simulink model "Simulation"  (R2018a)
settings: Solver=VariableStepAuto  StartTime=0.0  StopTime=10  FixedStep=1e-6  MaxStep=Tsc  RelTol=1e-3  EnableMultiTasking=on
InitFcn:
  | clc
  | close all
  | clear all
  | 
  | %Vector-space-decomposition transform (2)
  | D = 2/6*[cos(0) cos(1*pi/3) cos(2*pi/3) cos(3*pi/3) cos(4*pi/3) cos(5*pi/3);
  |         sin(0) sin(1*pi/3) sin(2*pi/3) sin(3*pi/3) sin(4*pi/3) sin(5*pi/3);
  |         cos(2*0) cos(2*pi/3) cos(4*pi/3) cos(6*pi/3) cos(8*pi/3) cos(10*pi/3);
  |         sin(2*0) sin(2*pi/3) sin(4*pi/3) sin(6*pi/3) sin(8*pi/3) sin(10*pi/3);
  |         1/2 1/2  1/2 1/2 1/2 1/2;
  |         1/2 -1/2 1/2 -1/2 1/2 -1/2];
  | 
  | %Control sampling period
  | Tsc = 1e-4;
  | 
  | %Parameters of six-phase induction machine (other than stator resistance):
  | P=2; %Number of machine pole pairs
  | Lm=284e-3; %alpha-beta magnetizing inductance (mH)
  | Rr=2.9; %alpha-beta rotor resistance (ohm)
  | Lls=10e-3; %alpha-beta stator leakage inductance (mH)
  | Llr=21e-3; %alpha-beta rotor leakage inductance (mH)
  | Lxy=4.52e-3; %xy stator inductance (mH)
  | L0=24.5e-3; %0- stator inductance (mH)
  | J=0.0261; %Inertia (Kg*m^2)
  | f=0.0033; %Friction coefficient (N*m*s)
  | Ls = Lls+Lm; Lr = Llr+Lm;  %alpha-beta self-inductances (mH)
undefined symbols (not defined in the file): DiscIntNeverNeededParam
libraries: powerlib x37, simulink x20, simulink_extras x7
(part 1 of 3)
settings Model: Creator=ayman.abdel-khalik  LastModifiedBy=agyepes
settings DataIOCC: LimitDataPoints=on  SaveFormat=Array
settings OptimizationCC: LifeSpan=inf
settings DebuggingCC: SolverPrmCheckMsg=warning  AllowSymbolicDim=off  SFUnexpectedBacktrackingDiag=warning  SFNoUnconditionalDefaultTransitionDiag=warning  SFExecutionAtInitializationDiag=none
settings HardwareCC: ProdBitPerPointer=32  ProdBitPerSizeT=32  ProdBitPerPtrDiffT=32  ProdLargestAtomicFloat=None  ProdIntDivRoundTo=Undefined  ProdEndianess=Unspecified  ProdWordSize=32  ProdHWDeviceType=32-bit Generic
settings ModelReferenceCC: PropagateSignalLabelsOutOfModel=off
settings CodeAppCC: StateflowObjectComments=on
settings GRTTargetCC: TargetLangStandard=C89/C90 (ANSI)
settings ConfigComp: CovMetricSettings=dw  CovSaveCumulativeToWorkspaceVar=on  CovSaveSingleToWorkspaceVar=on  CovExternalEMLEnable=off  CovSFcnEnable=off
settings SimscapeCC: SimscapeNormalizeSystem=off

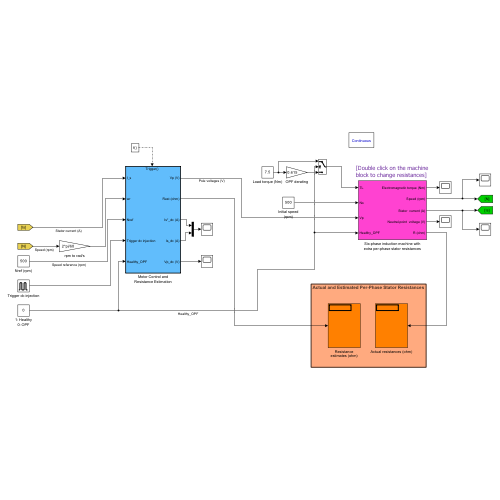
[thumbnail: Simulink's stored preview of the top-level diagram]
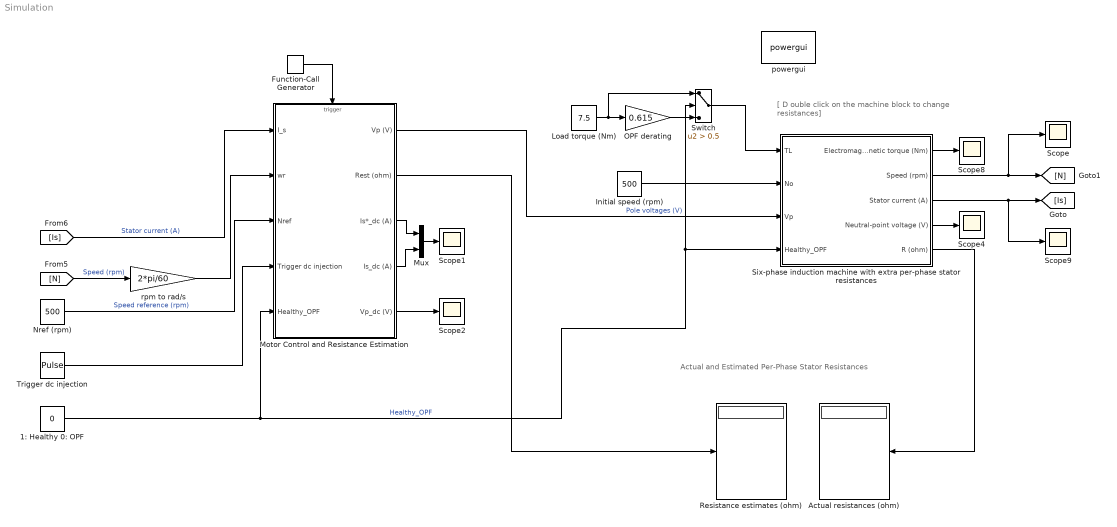
== system Simulation ==
  note: Actual and Estimated Per-Phase Stator Resistances
  note: [ D ouble click on the machine
      | block to change resistances]
  1: Healthy 0: OPF : Constant  Value=0
  Actual resistances (ohm) : Display
  Function-Call Generator : simulink/Ports & Subsystems/Function-Call Generator  sample_time=Tsc  numberOfIterations=1
  Initial speed (rpm) : Constant  Value=500
  Load torque (Nm) : Constant  Value=7.5
  Motor Control and Resistance Estimation : Subsystem
  Mux : Mux  Inputs=2
  Nref (rpm) : Constant  Value=500
  OPF derating : Gain  Gain=0.615
  Resistance estimates (ohm) : Display
  Scope{,1..2,4,8..9} (6 alike) : Scope
  Six-phase induction machine with extra per-phase stator resistances : Subsystem  mask{Radd=[3.15 5.1 2.15 4.4 0.2 0.05], Rs=4.4, Rr=Rr, Lm=Lm, Ls=Ls, Lr=Lr}
      mask prompts: Radd "Additional per-phase resistances [0-100] (ohm)"; Rs "Nominal stator resistance (ohm)"; Rr "Rotor resistance"; Lm "Alpha-beta magnetizing inductance"; Ls "Alpha-beta stator self-inductance"; Lr "Alpha-beta rotor self-inductance"
      mask init:
      | %In absence of extra resistances, the stator resistance is equal in all VSD
      | %subspaces:
      | Rxy = Rs;
      | R0 = Rs;
      | 
      | %Matrices for the machine alpha-beta equivalent circuit:
      | R1 = diag([Rs Rs Rr Rr]);
      | L1 = [Ls 0 Lm 0;
      | 	  0 Ls 0 Lm;
      | 	  Lm 0 Lr 0;
      | 	  0 Lm 0 Lr];
      | G1 = [0 0 0 0;
      |     0 0 0 0;
      |     0 0 0 1;
      |     0 0 -1 0];
      | 
      | L2=[0 0 Lm 0;
      | 	  0 0 0 Lm;
      | 	  0 0 0 0];
  Switch : Switch  Criteria=u2 > Threshold  Threshold=0.5
  Trigger dc injection : DiscretePulseGenerator  PulseType=Time based  Period=360  PhaseDelay=2
  powergui : powerlib/powergui  Priority=1  SimulationMode=Continuous  SampleTime=1e-4  frequency=60  Iterations=50  frequencyindice=0  Pbase=100e6  ErrMax=1e-4  UnitsV=kV  UnitsW=MW  buscounter=0  FunctionMessages=off  echomessages=off  EnableUseOfTLC=off  CurrentSourceSwitches=off  DisableSnubberDevices=off  DisableRonSwitches=off  DisableVfSwitches=off  DisplayEquations=off  AutomaticDiscreteSolvers=off  SolverType=Tustin/Backward Euler (TBE)  Interpol=off  ExternalGateDelay=off  methode=off  Ts=100  x0status=blocks  SPID=off  SwTol=0  HookPort=off  NonlinearTolerance=1e-4  nMaxIteration=100  ContinueOnMaxIteration=off  RestoreLinks=warning  ResistiveCurrentMeasurement=off  Frange=[0:2:500]  Ylog=off  Xlog=on  ShowGrid=off  save=off  variable=ZData  structure=0  ZoomFFT=off  StartTime=0.0  cycles=1  DisplayStyle=1  fundamental=60  FreqAxis=off  MaxFrequency=1000  frequencyindicesteady=1  RmsSteady=1  display=off
  rpm to rad/s : Gain  Gain=2*pi/60
  wires:
  [N] -> rpm to rad/s/1  "Speed (rpm)"
  [Is] -> Motor Control and Resistance Estimation/1(I_s)  "Stator current (A)"
  rpm to rad/s/1 -> Motor Control and Resistance Estimation/2(wr)
  Nref (rpm)/1 -> Motor Control and Resistance Estimation/3(Nref)  "Speed reference (rpm)"
  Motor Control and Resistance Estimation/1(Vp (V)) -> Six-phase induction machine with extra per-phase stator resistances/3(Vp)  "Pole voltages (V)"
  Motor Control and Resistance Estimation/2(Rest (ohm)) -> Resistance estimates (ohm)/1
  Trigger dc injection/1 -> Motor Control and Resistance Estimation/4(Trigger dc injection)
  Function-Call Generator/1 -> Motor Control and Resistance Estimation/Trigger
  Six-phase induction machine with extra per-phase stator resistances/2(Speed (rpm)) -> Scope/1, [N]
  Six-phase induction machine with extra per-phase stator resistances/3(Stator current (A)) -> Scope9/1, [Is]
  Switch/1 -> Six-phase induction machine with extra per-phase stator resistances/1(TL)
  Initial speed (rpm)/1 -> Six-phase induction machine with extra per-phase stator resistances/2(No)
  Six-phase induction machine with extra per-phase stator resistances/1(Electromagnetic torque (Nm)) -> Scope8/1
  Six-phase induction machine with extra per-phase stator resistances/4(Neutral-point voltage (V)) -> Scope4/1
  Six-phase induction machine with extra per-phase stator resistances/5(R (ohm)) -> Actual resistances (ohm)/1
  1: Healthy 0: OPF/1 -> Switch/2, Six-phase induction machine with extra per-phase stator resistances/4(Healthy_OPF), Motor Control and Resistance Estimation/5(Healthy_OPF)  "Healthy_OPF"
  Load torque (Nm)/1 -> Switch/1, OPF derating/1
  OPF derating/1 -> Switch/3
  Motor Control and Resistance Estimation/3(Is*_dc (A)) -> Mux/1
  Motor Control and Resistance Estimation/4(Is_dc (A)) -> Mux/2
  Mux/1 -> Scope1/1
  Motor Control and Resistance Estimation/5(Vp_dc (V)) -> Scope2/1

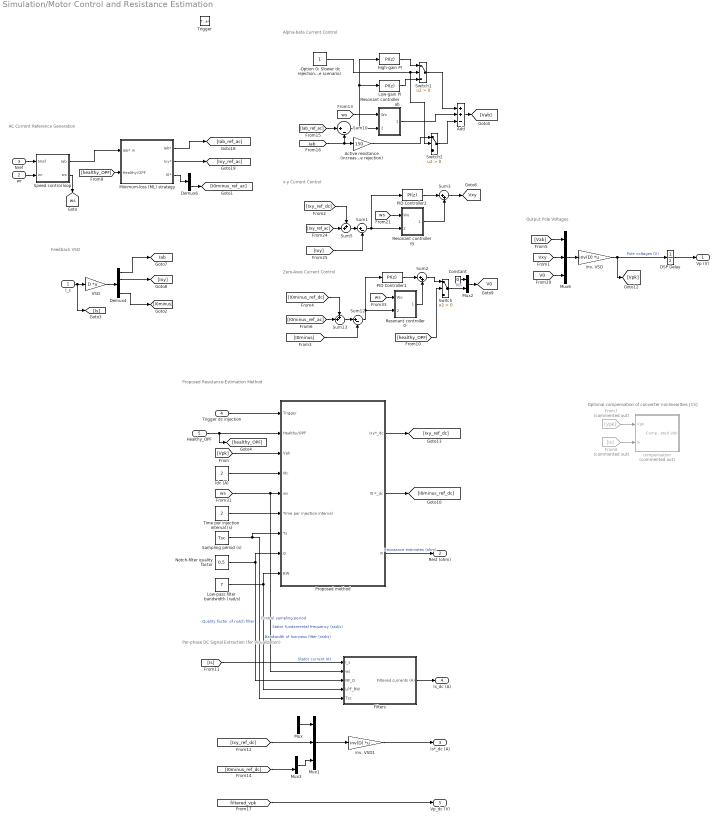
== system Simulation/Motor Control and Resistance Estimation ==
  note: Per-phase DC Signal Extraction (for Visualization)
  note: Optional compensation of converter nonlinearities [15]
  note: AC Current Reference Generation
  note: Output Pole Voltages
  note: Alpha-beta Current Control
  note: Feedback VSD
  note: x-y Current Control
  note: Zero-Axes Current Control
  note: Proposed Resistance-Estimation Method
  I_s : Inport
  wr : Inport  Port=2
  Nref : Inport  Port=3
  Trigger dc injection : Inport  Port=4
  Healthy_OPF : Inport  Port=5
  Trigger : TriggerPort  TriggerType=function-call  VariantControl=(inherit)  SampleTime=1e-4  PortDimensions=1
  "-Option 0: Slower dc rejection -Option 1: Faster dc rejection In experiments, 0 is used (worst-case scenario)" : Constant
  Active resistance (increases disturbance rejection) : Gain  Gain=150
  Add : Sum  Inputs=++-
  Constant : Constant  Value=0
  DSP Delay : UnitDelay  SampleTime=-1  HasFrameUpgradeWarning=on
  Demux4 : Demux  Outputs=[2 2 1 1 ]
  Demux6 : Demux  Outputs=2
  Filters : Subsystem
  From7 : From  Commented=on  GotoTag=Vpk
  From8 : From  Commented=on  GotoTag=Is
  High-gain PI : simulink/Continuous/PID Controller  Controller=PI  Form=Parallel  TimeDomain=Discrete-time  SampleTime=-1  IntegratorMethod=Forward Euler  ControllerParametersSource=internal  P=5  I=20000  D=0.001  N=100  UseFilter=on  TunerSelectOption=Transfer Function Based (PID Tuner App)  ZeroCross=off  InitialConditionSource=internal  InitialConditionForIntegrator=0  InitialConditionForFilter=0  DifferentiatorICPrevScaledInput=0  ExternalReset=none  TrackingMode=off  Kt=1  LimitOutput=on  UpperSaturationLimit=100  LowerSaturationLimit=-100  LinearizeAsGain=off  AntiWindupMode=clamping  Kb=1  POutMin=[]  POutMax=[]  IOutMin=[]  IOutMax=[]  DOutMin=[]  DOutMax=[]  NOutMin=[]  NOutMax=[]  SumOutMin=[]  SumOutMax=[]  SaturationOutMin=[]  SaturationOutMax=[]  PParamMin=[]  PParamMax=[]  IParamMin=[]  IParamMax=[]  DParamMin=[]  DParamMax=[]  NParamMin=[]  NParamMax=[]  KbParamMin=[]  KbParamMax=[]  KtParamMin=[]  KtParamMax=[]  KbOutMin=[]  KbOutMax=[]  KtOutMin=[]  KtOutMax=[]  IntegratorOutMin=[]  IntegratorOutMax=[]  FilterOutMin=[]  FilterOutMax=[]  SumI1OutMin=[]  SumI1OutMax=[]  SumI2OutMin=[]  SumI2OutMax=[]  SumI3OutMin=[]  SumI3OutMax=[]  SumDOutMin=[]  SumDOutMax=[]  DifferentiatorOutMin=[]  DifferentiatorOutMax=[]  FilterDiffOutCoefMin=[]  FilterDiffOutCoefMax=[]  ReciprocalOutMin=[]  ReciprocalOutMax=[]  SumDenOutMin=[]  SumDenOutMax=[]  SumNumOutMin=[]  SumNumOutMax=[]  DivideOutMin=[]  DivideOutMax=[]  IntegratorContinuousStateAttributes=''  IntegratorStateMustResolveToSignalObject=off  IntegratorRTWStateStorageClass=Auto  FilterContinuousStateAttributes=''  FilterStateMustResolveToSignalObject=off  FilterRTWStateStorageClass=Auto
  Idc (A) : Constant  Value=2
  Low-gain PI : simulink/Continuous/PID Controller  Controller=PI  Form=Parallel  TimeDomain=Discrete-time  SampleTime=-1  IntegratorMethod=Forward Euler  ControllerParametersSource=internal  P=2.6  I=670  D=0.001  N=100  UseFilter=on  TunerSelectOption=Transfer Function Based (PID Tuner App)  ZeroCross=off  InitialConditionSource=internal  InitialConditionForIntegrator=0  InitialConditionForFilter=0  DifferentiatorICPrevScaledInput=0  ExternalReset=none  TrackingMode=off  Kt=1  LimitOutput=on  UpperSaturationLimit=100  LowerSaturationLimit=-100  LinearizeAsGain=off  AntiWindupMode=clamping  Kb=1  POutMin=[]  POutMax=[]  IOutMin=[]  IOutMax=[]  DOutMin=[]  DOutMax=[]  NOutMin=[]  NOutMax=[]  SumOutMin=[]  SumOutMax=[]  SaturationOutMin=[]  SaturationOutMax=[]  PParamMin=[]  PParamMax=[]  IParamMin=[]  IParamMax=[]  DParamMin=[]  DParamMax=[]  NParamMin=[]  NParamMax=[]  KbParamMin=[]  KbParamMax=[]  KtParamMin=[]  KtParamMax=[]  KbOutMin=[]  KbOutMax=[]  KtOutMin=[]  KtOutMax=[]  IntegratorOutMin=[]  IntegratorOutMax=[]  FilterOutMin=[]  FilterOutMax=[]  SumI1OutMin=[]  SumI1OutMax=[]  SumI2OutMin=[]  SumI2OutMax=[]  SumI3OutMin=[]  SumI3OutMax=[]  SumDOutMin=[]  SumDOutMax=[]  DifferentiatorOutMin=[]  DifferentiatorOutMax=[]  FilterDiffOutCoefMin=[]  FilterDiffOutCoefMax=[]  ReciprocalOutMin=[]  ReciprocalOutMax=[]  SumDenOutMin=[]  SumDenOutMax=[]  SumNumOutMin=[]  SumNumOutMax=[]  DivideOutMin=[]  DivideOutMax=[]  IntegratorContinuousStateAttributes=''  IntegratorStateMustResolveToSignalObject=off  IntegratorRTWStateStorageClass=Auto  FilterContinuousStateAttributes=''  FilterStateMustResolveToSignalObject=off  FilterRTWStateStorageClass=Auto
  Low-pass filter bandwidth (rad/s) : Constant  Value=7
  Minimum-loss (ML) strategy : Subsystem
  Mux : Mux  Inputs=2
  Mux1 : Mux  Inputs=3
  Mux2 : Mux  Inputs=2
  Mux3 : Mux  Inputs=2
  Mux6 : Mux  Inputs=3
  Notch-filter quality factor : Constant  Value=0.5
  PID Controller1 : simulink/Continuous/PID Controller  Controller=PI  Form=Parallel  TimeDomain=Discrete-time  SampleTime=-1  IntegratorMethod=Forward Euler  ControllerParametersSource=internal  P=1.6  I=670  D=0.001  N=100  UseFilter=on  TunerSelectOption=Transfer Function Based (PID Tuner App)  ZeroCross=off  InitialConditionSource=internal  InitialConditionForIntegrator=0  InitialConditionForFilter=0  DifferentiatorICPrevScaledInput=0  ExternalReset=none  TrackingMode=off  Kt=1  LimitOutput=on  UpperSaturationLimit=100  LowerSaturationLimit=-100  LinearizeAsGain=off  AntiWindupMode=clamping  Kb=1  POutMin=[]  POutMax=[]  IOutMin=[]  IOutMax=[]  DOutMin=[]  DOutMax=[]  NOutMin=[]  NOutMax=[]  SumOutMin=[]  SumOutMax=[]  SaturationOutMin=[]  SaturationOutMax=[]  PParamMin=[]  PParamMax=[]  IParamMin=[]  IParamMax=[]  DParamMin=[]  DParamMax=[]  NParamMin=[]  NParamMax=[]  KbParamMin=[]  KbParamMax=[]  KtParamMin=[]  KtParamMax=[]  KbOutMin=[]  KbOutMax=[]  KtOutMin=[]  KtOutMax=[]  IntegratorOutMin=[]  IntegratorOutMax=[]  FilterOutMin=[]  FilterOutMax=[]  SumI1OutMin=[]  SumI1OutMax=[]  SumI2OutMin=[]  SumI2OutMax=[]  SumI3OutMin=[]  SumI3OutMax=[]  SumDOutMin=[]  SumDOutMax=[]  DifferentiatorOutMin=[]  DifferentiatorOutMax=[]  FilterDiffOutCoefMin=[]  FilterDiffOutCoefMax=[]  ReciprocalOutMin=[]  ReciprocalOutMax=[]  SumDenOutMin=[]  SumDenOutMax=[]  SumNumOutMin=[]  SumNumOutMax=[]  DivideOutMin=[]  DivideOutMax=[]  IntegratorContinuousStateAttributes=''  IntegratorStateMustResolveToSignalObject=off  IntegratorRTWStateStorageClass=Auto  FilterContinuousStateAttributes=''  FilterStateMustResolveToSignalObject=off  FilterRTWStateStorageClass=Auto
  PID Controller2 : simulink/Continuous/PID Controller  Controller=PI  Form=Parallel  TimeDomain=Discrete-time  SampleTime=-1  IntegratorMethod=Forward Euler  ControllerParametersSource=internal  P=1.6  I=670  D=0.001  N=100  UseFilter=on  TunerSelectOption=Transfer Function Based (PID Tuner App)  ZeroCross=off  InitialConditionSource=internal  InitialConditionForIntegrator=0  InitialConditionForFilter=0  DifferentiatorICPrevScaledInput=0  ExternalReset=none  TrackingMode=off  Kt=1  LimitOutput=on  UpperSaturationLimit=100  LowerSaturationLimit=-100  LinearizeAsGain=off  AntiWindupMode=clamping  Kb=1  POutMin=[]  POutMax=[]  IOutMin=[]  IOutMax=[]  DOutMin=[]  DOutMax=[]  NOutMin=[]  NOutMax=[]  SumOutMin=[]  SumOutMax=[]  SaturationOutMin=[]  SaturationOutMax=[]  PParamMin=[]  PParamMax=[]  IParamMin=[]  IParamMax=[]  DParamMin=[]  DParamMax=[]  NParamMin=[]  NParamMax=[]  KbParamMin=[]  KbParamMax=[]  KtParamMin=[]  KtParamMax=[]  KbOutMin=[]  KbOutMax=[]  KtOutMin=[]  KtOutMax=[]  IntegratorOutMin=[]  IntegratorOutMax=[]  FilterOutMin=[]  FilterOutMax=[]  SumI1OutMin=[]  SumI1OutMax=[]  SumI2OutMin=[]  SumI2OutMax=[]  SumI3OutMin=[]  SumI3OutMax=[]  SumDOutMin=[]  SumDOutMax=[]  DifferentiatorOutMin=[]  DifferentiatorOutMax=[]  FilterDiffOutCoefMin=[]  FilterDiffOutCoefMax=[]  ReciprocalOutMin=[]  ReciprocalOutMax=[]  SumDenOutMin=[]  SumDenOutMax=[]  SumNumOutMin=[]  SumNumOutMax=[]  DivideOutMin=[]  DivideOutMax=[]  IntegratorContinuousStateAttributes=''  IntegratorStateMustResolveToSignalObject=off  IntegratorRTWStateStorageClass=Auto  FilterContinuousStateAttributes=''  FilterStateMustResolveToSignalObject=off  FilterRTWStateStorageClass=Auto
  Proposed method : Subsystem
  Resonant controller 0- : Subsystem
  Resonant controller ab : Subsystem
  Resonant controller xy : Subsystem
  Sampling period (s) : Constant  Value=Tsc
  Speed control loop : Subsystem
  Sum1 : Sum  Inputs=|+-
  Sum10 : Sum  Inputs=|+-
  Sum12 : Sum  Inputs=|+-
  Sum13 : Sum  Inputs=++|
  Sum2 : Sum  Inputs=|++
  Sum3 : Sum  Inputs=|++
  Sum5 : Sum  Inputs=++|
  Switch : Switch  Criteria=u2 > Threshold
  Switch1 : Switch  Criteria=u2 > Threshold
  Switch2 : Switch  Criteria=u2 > Threshold
  Time per injection interval (s) : Constant  Value=2
  VSD : Gain  Gain=D  Multiplication=Matrix(K*u)
  compensation : Subsystem  Commented=on  mask{VDC=300, TPWM=Tsc, DT0=380e-9, ton=750e-9, toff=900e-9}
      mask prompts: VDC "Dc-link voltage (V)"; TPWM "Switching period (s)"; DT0 "Dead time (s)"; ton "Turn-on time (s)"; toff "Turn-off time (s)"
      mask init:
      | DT=DT0/TPWM;
      | Dly=(toff-ton)/TPWM;
  inv. VSD : Gain  Gain=inv(D)  Multiplication=Matrix(K*u)
  inv. VSD1 : Gain  Gain=inv(D)  Multiplication=Matrix(K*u)
  Vp (V) : Outport
  Rest (ohm) : Outport  Port=2
  Is*_dc (A) : Outport  Port=3
  Is_dc (A) : Outport  Port=4
  Vp_dc (V) : Outport  Port=5
  tag scope: Iab=global, V0=global, Vxy=global, ws=global
  wires:
  [Iab] -> Active resistance (increases disturbance rejection)/1, Sum10/2
  Sum10/1 -> Low-gain PI/1, High-gain PI/1, Resonant controller ab/2(error)
  [ws] -> Resonant controller ab/1(Wo)
  Add/1 -> [Vab]
  Mux6/1 -> inv. VSD/1
  wr/1 -> Speed control loop/2(wr)
  Nref/1 -> Speed control loop/1(Nref)
  inv. VSD/1 -> DSP Delay/1, [Vpk]  "Pole voltages (V)"
  [Vxy] -> Mux6/2
  [V0] -> Mux6/3
  [Vab] -> Mux6/1
  Demux4/4 -> [I0minus]
  Demux4/2 -> [Ixy]
  I_s/1 -> [Is], VSD/1
  Demux4/1 -> [Iab]
  VSD/1 -> Demux4/1
  Speed control loop/2(ws) -> [ws]
  Speed control loop/1(Iab) -> Minimum-loss (ML) strategy/1(Iab* in)
  Demux6/2 -> [I0minus_ref_ac]
  Minimum-loss (ML) strategy/1(Iab*) -> [Iab_ref_ac]
  Minimum-loss (ML) strategy/2(Ixy*) -> [Ixy_ref_ac]
  Minimum-loss (ML) strategy/3(I0*) -> Demux6/1
  Sum5/1 -> Sum1/1
  [ws] -> Resonant controller xy/1(Wo)
  PID Controller2/1 -> Sum3/1
  [Ixy] -> Sum1/2
  [Ixy_ref_dc] -> Sum5/1
  Sum1/1 -> Resonant controller xy/2(error), PID Controller2/1
  Sum3/1 -> [Vxy]
  Mux2/1 -> [V0]
  Sum13/1 -> Sum12/1
  [I0minus_ref_dc] -> Sum13/1
  Sum12/1 -> Resonant controller 0-/2(error), PID Controller1/1
  [I0minus] -> Sum12/2
  [ws] -> Resonant controller 0-/1(Wo)
  From7/1 -> compensation/1(Vpk)
  From8/1 -> compensation/2(Is)
  [Vpk] -> Proposed method/3(Vpk)
  [Iab_ref_ac] -> Sum10/1
  Resonant controller ab/1(Vref) -> Add/2
  Resonant controller xy/1(Vref) -> Sum3/2
  PID Controller1/1 -> Sum2/1
  Resonant controller 0-/1(Vref) -> Sum2/2
  Switch/1 -> Mux2/2  "V0-"
  Healthy_OPF/1 -> [healthy_OPF], Proposed method/2(Healthy/OPF)
  Proposed method/1(Ixy*_dc) -> [Ixy_ref_dc]
  Trigger dc injection/1 -> Proposed method/1(Trigger)
  Proposed method/2(I0-*_dc) -> [I0minus_ref_dc]
  Proposed method/3("R ") -> Rest (ohm)/1  "Resistance estimates (ohm)"
  [Ixy_ref_ac] -> Sum5/2
  DSP Delay/1 -> Vp (V)/1
  [I0minus_ref_ac] -> Sum13/2
  Idc (A)/1 -> Proposed method/4(Idc)
  Time per injection interval (s)/1 -> Proposed method/6(Time per injection interval)
  [healthy_OPF] -> Minimum-loss (ML) strategy/2(Healthy/OPF)
  Constant/1 -> Mux2/1
  [healthy_OPF] -> Switch/2
  Sum2/1 -> Switch/1
  Switch1/1 -> Add/1
  Switch2/1 -> Add/3
  High-gain PI/1 -> Switch1/1
  Active resistance (increases disturbance rejection)/1 -> Switch2/1
  "-Option 0: Slower dc rejection -Option 1: Faster dc rejection In experiments, 0 is used (worst-case scenario)"/1 -> Switch2/2, Switch1/2
  Low-gain PI/1 -> Switch1/3
  [Is] -> Filters/1(I_s)  "Stator current (A)"
  [ws] -> Filters/2(ws), Proposed method/5(ws)  "Stator fundamental frequency (rad/s)"
  Notch-filter quality factor/1 -> Filters/3(NF_Q), Proposed method/8(Q)  "Quality factor of notch filter"
  Low-pass filter bandwidth (rad/s)/1 -> Filters/4(LPF_BW), Proposed method/9(BW)  "Bandwidth of low-pass filter (rad/s)"
  Sampling period (s)/1 -> Filters/5(Tsc), Proposed method/7(Ts)  "Control sampling period"
  [Ixy_ref_dc] -> Mux1/2
  Mux/1 -> Mux1/1
  Mux1/1 -> inv. VSD1/1
  [I0minus_ref_dc] -> Mux3/2
  Mux3/1 -> Mux1/3
  Filters/1(Filtered currents (A)) -> Is_dc (A)/1
  inv. VSD1/1 -> Is*_dc (A)/1
  [filtered_vpk] -> Vp_dc (V)/1

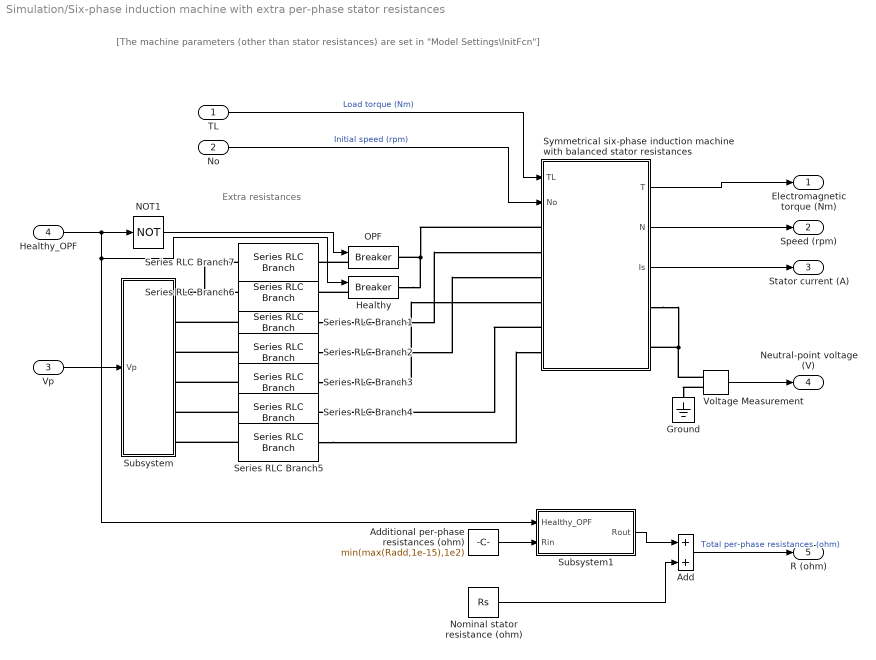
== system Simulation/Six-phase induction machine with extra per-phase stator resistances ==
  note: [The machine parameters (other than stator resistances) are set in "Model Settings\InitFcn"]
  note: Extra resistances
  TL : Inport
  No : Inport  Port=2
  Vp : Inport  Port=3
  Healthy_OPF : Inport  Port=4
  Add : Sum
  Additional per-phase resistances (ohm) : Constant  Value=min(max(Radd,1e-15),1e2)
  Ground : powerlib/Elements/Ground  LConnTagsString=a
  Healthy : powerlib/Elements/Breaker  InitialState=1  SwitchingTimes="[1/60  5/60]"  External=on  BreakerResistance=0  SnubberResistance=1e6  SnubberCapacitance=inf  Measurements=None  MoreParameters=on  NoBreakLoop=off
  NOT1 : Logic  Operator=NOT  IconShape=distinctive  AllPortsSameDT=off  OutDataTypeStr=boolean
  Nominal stator resistance (ohm) : Constant  Value=Rs
  OPF : powerlib/Elements/Breaker  InitialState=0  SwitchingTimes="[1/60  5/60]"  External=on  BreakerResistance=0  SnubberResistance=1e6  SnubberCapacitance=inf  Measurements=None  MoreParameters=on  NoBreakLoop=off
  Series RLC Branch1 : powerlib/Elements/Series RLC Branch  LConnTagsString=__new0  RConnTagsString=__new0  BranchType=R  Resistance=min(max(Radd(2),1e-15),1e2)  Inductance=1e-3  SetiL0=off  InitialCurrent=0  Capacitance=1e-6  Setx0=off  InitialVoltage=0  Measurements=None
  Series RLC Branch2 : powerlib/Elements/Series RLC Branch  LConnTagsString=__new0  RConnTagsString=__new0  BranchType=R  Resistance=min(max(Radd(3),1e-15),1e2)  Inductance=1e-3  SetiL0=off  InitialCurrent=0  Capacitance=1e-6  Setx0=off  InitialVoltage=0  Measurements=None
  Series RLC Branch3 : powerlib/Elements/Series RLC Branch  LConnTagsString=__new0  RConnTagsString=__new0  BranchType=R  Resistance=max(Radd(4),1e-15)  Inductance=1e-3  SetiL0=off  InitialCurrent=0  Capacitance=1e-6  Setx0=off  InitialVoltage=0  Measurements=None
  Series RLC Branch4 : powerlib/Elements/Series RLC Branch  LConnTagsString=__new0  RConnTagsString=__new0  BranchType=R  Resistance=min(max(Radd(5),1e-15),1e2)  Inductance=1e-3  SetiL0=off  InitialCurrent=0  Capacitance=1e-6  Setx0=off  InitialVoltage=0  Measurements=None
  Series RLC Branch5 : powerlib/Elements/Series RLC Branch  LConnTagsString=__new0  RConnTagsString=__new0  BranchType=R  Resistance=min(max(Radd(6),1e-15),1e2)  Inductance=1e-3  SetiL0=off  InitialCurrent=0  Capacitance=1e-6  Setx0=off  InitialVoltage=0  Measurements=None
  Series RLC Branch6 : powerlib/Elements/Series RLC Branch  LConnTagsString=__new0  RConnTagsString=__new0  BranchType=R  Resistance=min(max(Radd(1),1e-15),1e2)  Inductance=1e-3  SetiL0=off  InitialCurrent=0  Capacitance=1e-6  Setx0=off  InitialVoltage=0  Measurements=None
  Series RLC Branch7 : powerlib/Elements/Series RLC Branch  LConnTagsString=__new0  RConnTagsString=__new0  BranchType=R  Resistance=1e9  Inductance=1e-3  SetiL0=off  InitialCurrent=0  Capacitance=1e-6  Setx0=off  InitialVoltage=0  Measurements=None
  Subsystem : Subsystem
  Subsystem1 : Subsystem
  Symmetrical six-phase induction machine with balanced stator resistances : Subsystem
  Voltage Measurement : powerlib/Measurements/Voltage Measurement  PhasorSimulation=off  OutputType=Complex  PSBequivalent=0
  Electromagnetic torque (Nm) : Outport
  Speed (rpm) : Outport  Port=2
  Stator current (A) : Outport  Port=3
  Neutral-point voltage (V) : Outport  Port=4
  R (ohm) : Outport  Port=5
  wires:
  Symmetrical six-phase induction machine with balanced stator resistances/3(Is) -> Stator current (A)/1
  Voltage Measurement/1 -> Neutral-point voltage (V)/1
  Vp/1 -> Subsystem/1(Vp)
  Symmetrical six-phase induction machine with balanced stator resistances/1(T) -> Electromagnetic torque (Nm)/1
  TL/1 -> Symmetrical six-phase induction machine with balanced stator resistances/1(TL)  "Load torque (Nm)"
  No/1 -> Symmetrical six-phase induction machine with balanced stator resistances/2(No)  "Initial speed (rpm)"
  Symmetrical six-phase induction machine with balanced stator resistances/2(N) -> Speed (rpm)/1
  Nominal stator resistance (ohm)/1 -> Add/2
  Add/1 -> R (ohm)/1  "Total per-phase resistances (ohm)"
  NOT1/1 -> OPF/1
  Healthy_OPF/1 -> Subsystem1/1(Healthy_OPF), Healthy/1, NOT1/1
  Additional per-phase resistances (ohm)/1 -> Subsystem1/2(Rin)
  Subsystem1/1(Rout) -> Add/1
  connections:
  Series RLC Branch1/RConn1 -- Symmetrical six-phase induction machine with balanced stator resistances/LConn2
  Series RLC Branch2/LConn1 -- Subsystem/RConn3
  Series RLC Branch3/LConn1 -- Subsystem/RConn4
  Series RLC Branch3/RConn1 -- Symmetrical six-phase induction machine with balanced stator resistances/LConn4
  Symmetrical six-phase induction machine with balanced stator resistances/RConn1 -- Symmetrical six-phase induction machine with balanced stator resistances/RConn2 -- Voltage Measurement/LConn1
  Series RLC Branch4/LConn1 -- Subsystem/RConn5
  Symmetrical six-phase induction machine with balanced stator resistances/LConn5 -- Series RLC Branch4/RConn1
  Series RLC Branch5/RConn1 -- Symmetrical six-phase induction machine with balanced stator resistances/LConn6
  Series RLC Branch2/RConn1 -- Symmetrical six-phase induction machine with balanced stator resistances/LConn3
  Series RLC Branch1/LConn1 -- Subsystem/RConn2
  Voltage Measurement/LConn2 -- Ground/LConn1
  Series RLC Branch6/LConn1 -- Series RLC Branch7/LConn1 -- Subsystem/RConn1
  Series RLC Branch5/LConn1 -- Subsystem/RConn6
  OPF/LConn1 -- Series RLC Branch7/RConn1
  Healthy/LConn1 -- Series RLC Branch6/RConn1
  Symmetrical six-phase induction machine with balanced stator resistances/LConn1 -- Healthy/RConn1 -- OPF/RConn1

== system Simulation/Motor Control and Resistance Estimation/Filters ==
  I_s : Inport
  ws : Inport  Port=2
  NF_Q : Inport  Port=3
  LPF_BW : Inport  Port=4
  Tsc : Inport  Port=5
  Low-pass filter : Subsystem
  Notch filter : Subsystem
  Filtered currents (A) : Outport
  wires:
  NF_Q/1 -> Notch filter/4(Q)
  I_s/1 -> Low-pass filter/1(Vpk)
  Tsc/1 -> Notch filter/3(Tsc)
  ws/1 -> Notch filter/2(ws)
  LPF_BW/1 -> Low-pass filter/2(BW)
  Low-pass filter/1(Out) -> Notch filter/1(In)
  Notch filter/1(Out) -> Filtered currents (A)/1

== system Simulation/Motor Control and Resistance Estimation/Minimum-loss (ML) strategy ==
  Iab* in : Inport
  Healthy/OPF : Inport  Port=2
  K0_f : Gain  Gain=[0 0; -0.3333333 0]  Multiplication=Matrix(K*u)
  K0_h : Gain  Gain=[0 0; 0 0]  Multiplication=Matrix(K*u)
  Kab : Gain  Gain=[1 0;0 1]  Multiplication=Matrix(K*u)
  Kxy_f : Gain  Gain=[-0.66667 0; 0 0]  Multiplication=Matrix(K*u)
  Kxy_h : Gain  Gain=[0 0; 0 0]  Multiplication=Matrix(K*u)
  Switch : Switch  Criteria=u2 > Threshold
  Switch1 : Switch  Criteria=u2 > Threshold
  Iab* : Outport
  Ixy* : Outport  Port=2
  I0* : Outport  Port=3
  wires:
  Switch/1 -> I0*/1
  Kab/1 -> Iab*/1
  Kxy_f/1 -> Switch1/3  "OPF"
  Iab* in/1 -> Kab/1, Kxy_h/1, K0_h/1, K0_f/1, Kxy_f/1
  K0_f/1 -> Switch/3  "OPF"
  K0_h/1 -> Switch/1  "Healthy"
  Kxy_h/1 -> Switch1/1  "Healthy"
  Switch1/1 -> Ixy*/1
  Healthy/OPF/1 -> Switch1/2, Switch/2

== system Simulation/Motor Control and Resistance Estimation/Proposed method ==
  Trigger : Inport
  Healthy/OPF : Inport  Port=2
  Vpk : Inport  Port=3
  Idc : Inport  Port=4
  ws : Inport  Port=5
  Time per injection interval : Inport  Port=6
  Ts : Inport  Port=7
  Q : Inport  Port=8
  BW : Inport  Port=9
  Detect rising edge : Subsystem
  Generation of time sequence for injection : Subsystem
  R estimation : Subsystem
  dc current reference generation : Subsystem
  Ixy*_dc : Outport
  I0-*_dc : Outport  Port=2
  "R " : Outport  Port=3
  wires:
  Q/1 -> R estimation/3(NF_Q)
  Detect rising edge/1(Out) -> Generation of time sequence for injection/1(In)
  Idc/1 -> dc current reference generation/1(Idc), R estimation/6(Idc)
  Time per injection interval/1 -> Generation of time sequence for injection/2(interval)
  Generation of time sequence for injection/2(injecting) -> dc current reference generation/3(injecting)
  Healthy/OPF/1 -> dc current reference generation/2(Healthy/OPF), R estimation/7(Healthy/OPF)
  Generation of time sequence for injection/1(time_sequence) -> dc current reference generation/4(time_sequence)
  BW/1 -> R estimation/4(LPF_BW)
  Ts/1 -> R estimation/5(Tsc), Generation of time sequence for injection/3(Tsc)
  R estimation/1("R ") -> "R "/1
  dc current reference generation/1(Ixy*_dc) -> Ixy*_dc/1
  Vpk/1 -> R estimation/1(Vpk)  "Pole voltages (V)"
  dc current reference generation/2(I0-*_dc) -> I0-*_dc/1
  Trigger/1 -> Detect rising edge/1(In)
  ws/1 -> R estimation/2(ws)  "Stator fundamental frequency (rad/s)"

== system Simulation/Motor Control and Resistance Estimation/Resonant controller 0- ==
  Wo : Inport
  error : Inport  Port=2
  Adaptive Impulse invariant : Subsystem
  Kr : Gain  Gain=1650
  Vref : Outport
  wires:
  Kr/1 -> Adaptive Impulse invariant/1(in)
  error/1 -> Kr/1
  Wo/1 -> Adaptive Impulse invariant/2(Wo)
  Adaptive Impulse invariant/1(out) -> Vref/1

== system Simulation/Motor Control and Resistance Estimation/Resonant controller ab ==
  Wo : Inport
  error : Inport  Port=2
  Adaptive Impulse invariant : Subsystem
  Kr : Gain  Gain=14130
  Vref : Outport
  wires:
  Kr/1 -> Adaptive Impulse invariant/1(in)
  error/1 -> Kr/1
  Wo/1 -> Adaptive Impulse invariant/2(Wo)
  Adaptive Impulse invariant/1(out) -> Vref/1

== system Simulation/Motor Control and Resistance Estimation/Resonant controller xy ==
  Wo : Inport
  error : Inport  Port=2
  Adaptive Impulse invariant : Subsystem
  Kr : Gain  Gain=1650
  Vref : Outport
  wires:
  Adaptive Impulse invariant/1(out) -> Vref/1
  Wo/1 -> Adaptive Impulse invariant/2(Wo)
  error/1 -> Kr/1
  Kr/1 -> Adaptive Impulse invariant/1(in)

== system Simulation/Motor Control and Resistance Estimation/Speed control loop ==
  Nref : Inport
  wr : Inport  Port=2
  PI speed controller : simulink/Continuous/PID Controller  Controller=PI  Form=Parallel  TimeDomain=Discrete-time  SampleTime=-1  IntegratorMethod=Forward Euler  ControllerParametersSource=internal  P=0.12565  I=0.295  D=0  N=100  UseFilter=on  TunerSelectOption=Transfer Function Based (PID Tuner App)  InitialConditionSource=internal  InitialConditionForIntegrator=0  InitialConditionForFilter=0  DifferentiatorICPrevScaledInput=0  ExternalReset=none  TrackingMode=off  Kt=1  LimitOutput=on  UpperSaturationLimit=5  LowerSaturationLimit=-5  LinearizeAsGain=on  AntiWindupMode=clamping  Kb=1  POutMin=[]  POutMax=[]  IOutMin=[]  IOutMax=[]  DOutMin=[]  DOutMax=[]  NOutMin=[]  NOutMax=[]  SumOutMin=[]  SumOutMax=[]  SaturationOutMin=[]  SaturationOutMax=[]  PParamMin=[]  PParamMax=[]  IParamMin=[]  IParamMax=[]  DParamMin=[]  DParamMax=[]  NParamMin=[]  NParamMax=[]  KbParamMin=[]  KbParamMax=[]  KtParamMin=[]  KtParamMax=[]  KbOutMin=[]  KbOutMax=[]  KtOutMin=[]  KtOutMax=[]  IntegratorOutMin=[]  IntegratorOutMax=[]  FilterOutMin=[]  FilterOutMax=[]  SumI1OutMin=[]  SumI1OutMax=[]  SumI2OutMin=[]  SumI2OutMax=[]  SumI3OutMin=[]  SumI3OutMax=[]  SumDOutMin=[]  SumDOutMax=[]  DifferentiatorOutMin=[]  DifferentiatorOutMax=[]  FilterDiffOutCoefMin=[]  FilterDiffOutCoefMax=[]  ReciprocalOutMin=[]  ReciprocalOutMax=[]  SumDenOutMin=[]  SumDenOutMax=[]  SumNumOutMin=[]  SumNumOutMax=[]  DivideOutMin=[]  DivideOutMax=[]  IntegratorContinuousStateAttributes=''  IntegratorStateMustResolveToSignalObject=off  IntegratorRTWStateStorageClass=Auto  FilterContinuousStateAttributes=''  FilterStateMustResolveToSignalObject=off  FilterRTWStateStorageClass=Auto
  Pole pairs : Gain  Gain=P
  Subsystem2 : Subsystem
  Sum1 : Sum  Inputs=|+-
  d-axis current reference (A) : Constant  Value=1.41
  rpm to rad/s : Gain  Gain=2*pi/60
  Iab : Outport
  ws : Outport  Port=2
  wires:
  Subsystem2/1(Iab) -> Iab/1  "alpha-beta stator current (A)"
  Subsystem2/2(ws) -> ws/1  "Stator frequency (rad/s)"
  Pole pairs/1 -> Subsystem2/3(wr)  "Electrical speed (rad/s)"
  rpm to rad/s/1 -> Sum1/1
  Sum1/1 -> PI speed controller/1
  wr/1 -> Sum1/2, Pole pairs/1  "Actual mechanical speed (rad/s)"
  Nref/1 -> rpm to rad/s/1
  d-axis current reference (A)/1 -> Subsystem2/1(Id*)
  PI speed controller/1 -> Subsystem2/2(Iq*)  "q-axis current reference (A)"

== system Simulation/Motor Control and Resistance Estimation/compensation ==
  Vpk : Inport
  Is : Inport  Port=2
  Demux2 : Demux  Outputs=6
  Demux3 : Demux  Outputs=6
  Mux1 : Mux  Inputs=6
  Per-phase nonlinearity comp. a : Subsystem
  Per-phase nonlinearity comp. b : Subsystem
  Per-phase nonlinearity comp. c : Subsystem
  Per-phase nonlinearity comp. d : Subsystem
  Per-phase nonlinearity comp. e : Subsystem
  Per-phase nonlinearity comp. f : Subsystem
  Compensated Vpk : Outport
  wires:
  Demux2/3 -> Per-phase nonlinearity comp. c/2(Is)
  Per-phase nonlinearity comp. d/1(Compensated Vpk) -> Mux1/4
  Demux3/5 -> Per-phase nonlinearity comp. e/1(Vpk)
  Per-phase nonlinearity comp. c/1(Compensated Vpk) -> Mux1/3
  Demux3/2 -> Per-phase nonlinearity comp. b/1(Vpk)
  Demux3/3 -> Per-phase nonlinearity comp. c/1(Vpk)
  Demux3/4 -> Per-phase nonlinearity comp. d/1(Vpk)
  Demux2/1 -> Per-phase nonlinearity comp. a/2(Is)
  Per-phase nonlinearity comp. e/1(Compensated Vpk) -> Mux1/5
  Demux3/6 -> Per-phase nonlinearity comp. f/1(Vpk)
  Per-phase nonlinearity comp. f/1(Compensated Vpk) -> Mux1/6
  Demux3/1 -> Per-phase nonlinearity comp. a/1(Vpk)
  Per-phase nonlinearity comp. b/1(Compensated Vpk) -> Mux1/2
  Demux2/2 -> Per-phase nonlinearity comp. b/2(Is)
  Demux2/6 -> Per-phase nonlinearity comp. f/2(Is)
  Per-phase nonlinearity comp. a/1(Compensated Vpk) -> Mux1/1
  Demux2/5 -> Per-phase nonlinearity comp. e/2(Is)
  Demux2/4 -> Per-phase nonlinearity comp. d/2(Is)
  Vpk/1 -> Demux3/1
  Mux1/1 -> Compensated Vpk/1
  Is/1 -> Demux2/1

== system Simulation/Six-phase induction machine with extra per-phase stator resistances/Subsystem ==
  Vp : Inport
  Demux : Demux  Outputs=6
  Ground : powerlib/Elements/Ground  LConnTagsString=a
  V{1..6} (6 alike) : powerlib/Electrical Sources/Controlled Voltage Source  Initialize=on  Source_Type=AC  Amplitude=0  Phase=0  Frequency=0  Measurements=None
  1 : PMIOPort  Side=Right
  2 : PMIOPort  Port=2  Side=Right
  3 : PMIOPort  Port=3  Side=Right
  4 : PMIOPort  Port=4  Side=Right
  5 : PMIOPort  Port=5  Side=Right
  6 : PMIOPort  Port=6  Side=Right
  wires:
  Demux/5 -> V5/1
  Demux/3 -> V3/1
  Demux/6 -> V6/1
  Vp/1 -> Demux/1
  Demux/2 -> V2/1
  Demux/1 -> V1/1
  Demux/4 -> V4/1
  connections:
  V1/RConn1 -- 1/RConn1
  V2/RConn1 -- 2/RConn1
  V4/RConn1 -- 4/RConn1
  V5/RConn1 -- 5/RConn1
  V1/LConn1 -- V2/LConn1 -- Ground/LConn1 -- V3/LConn1 -- V4/LConn1 -- V5/LConn1 -- V6/LConn1
  V3/RConn1 -- 3/RConn1
  6/RConn1 -- V6/RConn1

== system Simulation/Six-phase induction machine with extra per-phase stator resistances/Subsystem1 ==
  Healthy_OPF : Inport
  Rin : Inport  Port=2
  Constant : Constant  Value=Inf
  Demux : Demux  Outputs=[1 5]
  Mux2 : Mux  Inputs=2
  Switch : Switch  Criteria=u2 > Threshold  Threshold=0.5
  Rout : Outport
  wires:
  Mux2/1 -> Rout/1
  Demux/1 -> Switch/1
  Demux/2 -> Mux2/2
  Constant/1 -> Switch/3
  Switch/1 -> Mux2/1
  Rin/1 -> Demux/1
  Healthy_OPF/1 -> Switch/2

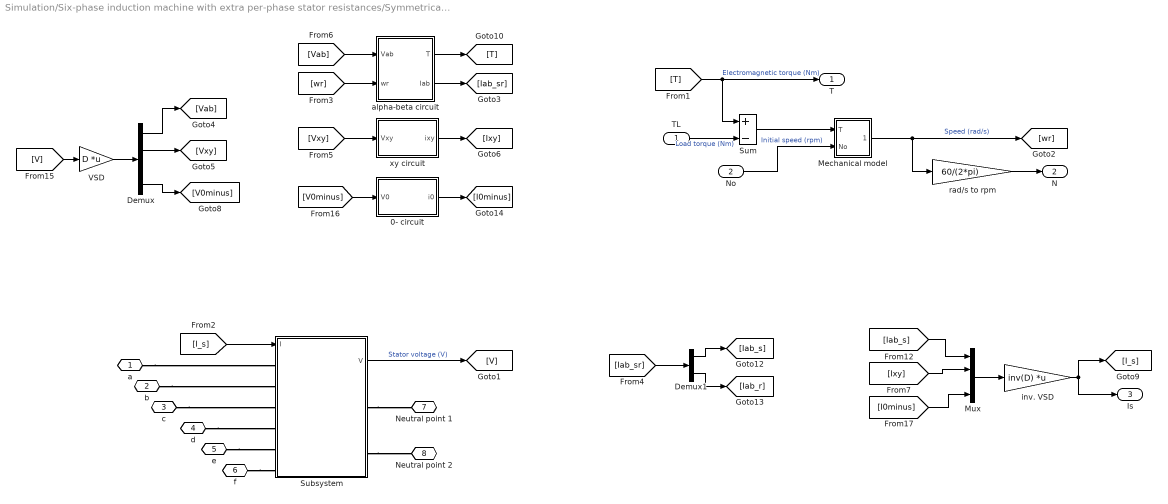
== system Simulation/Six-phase induction machine with extra per-phase stator resistances/Symmetrical six-phase induction machine with balanced stator resistances ==
  TL : Inport
  No : Inport  Port=2
  0- circuit : Subsystem
  Demux : Demux  Outputs=[2 2 1 1]
      settings: DisplayOption=none
  Demux1 : Demux  Outputs=[2 2]
      settings: DisplayOption=none
  Mechanical model : Subsystem
  Mux : Mux
  Subsystem : Subsystem
  Sum : Sum  Inputs=+-  InputSameDT=on  SaturateOnIntegerOverflow=on  OutDataTypeStr=Inherit: Same as first input
  VSD : Gain  Gain=D  Multiplication=Matrix(K*u)  SaturateOnIntegerOverflow=on  OutDataTypeStr=Inherit: Same as input  ParamDataTypeStr=Inherit: Same as input
  alpha-beta circuit : Subsystem
  inv. VSD : Gain  Gain=inv(D)  Multiplication=Matrix(K*u)  SaturateOnIntegerOverflow=on  OutDataTypeStr=Inherit: Same as input  ParamDataTypeStr=Inherit: Same as input
  rad/s to rpm : Gain  Gain=60/(2*pi)
  xy circuit : Subsystem
  a : PMIOPort  Side=Left
  b : PMIOPort  Port=2  Side=Left
  c : PMIOPort  Port=3  Side=Left
  d : PMIOPort  Port=4  Side=Left
  e : PMIOPort  Port=5  Side=Left
  f : PMIOPort  Port=6  Side=Left
  Neutral point 1 : PMIOPort  Port=7  Side=Right
  Neutral point 2 : PMIOPort  Port=8  Side=Right
  T : Outport  VectorParamsAs1DForOutWhenUnconnected=off
  N : Outport  Port=2  VectorParamsAs1DForOutWhenUnconnected=off
  Is : Outport  Port=3  VectorParamsAs1DForOutWhenUnconnected=off
  wires:
  VSD/1 -> Demux/1
  Mux/1 -> inv. VSD/1
  alpha-beta circuit/1(T) -> [T]
  [wr] -> alpha-beta circuit/2(wr)
  alpha-beta circuit/2(Iab) -> [Iab_sr]
  [Iab_sr] -> Demux1/1
  Demux/1 -> [Vab]
  Demux/2 -> [Vxy]
  [Ixy] -> Mux/2
  inv. VSD/1 -> Is/1, [I_s]
  Demux1/1 -> [Iab_s]
  Demux1/2 -> [Iab_r]
  [Iab_s] -> Mux/1
  [Vab] -> alpha-beta circuit/1(Vab)
  [I_s] -> Subsystem/1(I)
  [V] -> VSD/1
  rad/s to rpm/1 -> N/1
  Demux/4 -> [V0minus]
  [I0minus] -> Mux/4
  [Vxy] -> xy circuit/1(Vxy)
  xy circuit/1(ixy) -> [Ixy]
  [V0minus] -> 0- circuit/1(V0)
  0- circuit/1(i0) -> [I0minus]
  Mechanical model/1(wm) -> [wr], rad/s to rpm/1  "Speed (rad/s)"
  Subsystem/1(V) -> [V]  "Stator voltage (V)"
  Sum/1 -> Mechanical model/1(T)
  [T] -> Sum/1, T/1  "Electromagnetic torque (Nm)"
  TL/1 -> Sum/2  "Load torque (Nm)"
  No/1 -> Mechanical model/2(No)  "Initial speed (rpm)"
  connections:
  a/RConn1 -- Subsystem/LConn1
  b/RConn1 -- Subsystem/LConn2
  c/RConn1 -- Subsystem/LConn3
  d/RConn1 -- Subsystem/LConn4
  e/RConn1 -- Subsystem/LConn5
  f/RConn1 -- Subsystem/LConn6
  Subsystem/RConn1 -- Neutral point 1/RConn1
  Subsystem/RConn2 -- Neutral point 2/RConn1

== system Simulation/Motor Control and Resistance Estimation/Filters/Low-pass filter ==
  Vpk : Inport
  BW : Inport  Port=2
  Product : Product
  Product1 : Product
  Sum1 : Sum  Inputs=+-  SaturateOnIntegerOverflow=on
  Sum2 : Sum  Inputs=+-  SaturateOnIntegerOverflow=on
  integrator : DiscreteIntegrator  gainval=1  SampleTime=-1  ICPrevOutput=DiscIntNeverNeededParam  ICPrevScaledInput=DiscIntNeverNeededParam
  integrator2 : DiscreteIntegrator  gainval=1  SampleTime=-1  ICPrevOutput=DiscIntNeverNeededParam  ICPrevScaledInput=DiscIntNeverNeededParam
  Out : Outport
  wires:
  integrator/1 -> Sum2/1, Sum1/2
  integrator2/1 -> Out/1, Sum2/2
  Product/1 -> integrator/1
  Sum1/1 -> Product/2
  Sum2/1 -> Product1/2
  Product1/1 -> integrator2/1
  BW/1 -> Product/1, Product1/1
  Vpk/1 -> Sum1/1

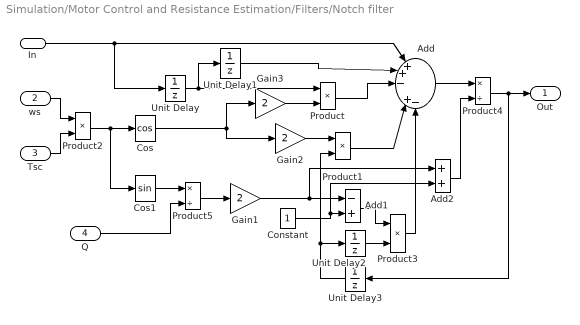
== system Simulation/Motor Control and Resistance Estimation/Filters/Notch filter ==
  In : Inport
  ws : Inport  Port=2
  Tsc : Inport  Port=3
  Q : Inport  Port=4
  Add : Sum  Inputs=|++-|+-
  Add1 : Sum  Inputs=-+
  Add2 : Sum
  Constant : Constant
  Cos : Trigonometry  Operator=cos
  Cos1 : Trigonometry
  Gain1 : Gain  Gain=2
  Gain2 : Gain  Gain=2
  Gain3 : Gain  Gain=2
  Product{,1..3} (4 alike) : Product
  Product4 : Product  Inputs=*/
  Product5 : Product  Inputs=*/
  Unit Delay{,1..3} (4 alike) : UnitDelay  SampleTime=-1  HasFrameUpgradeWarning=on
  Out : Outport
  wires:
  Product4/1 -> Out/1, Unit Delay3/1
  Add2/1 -> Product4/2
  Add/1 -> Product4/1
  Cos1/1 -> Product5/1
  Gain3/1 -> Product/2
  Product/1 -> Add/3
  Product3/1 -> Add/5
  ws/1 -> Product2/1
  Constant/1 -> Add1/2, Add2/2
  Unit Delay2/1 -> Product3/2
  Cos/1 -> Gain2/1, Gain3/1
  Product1/1 -> Add/4
  Unit Delay/1 -> Product/1, Unit Delay1/1
  In/1 -> Unit Delay/1, Add/1
  Unit Delay3/1 -> Product1/2, Unit Delay2/1
  Unit Delay1/1 -> Add/2
  Product2/1 -> Cos/1, Cos1/1
  Product5/1 -> Gain1/1
  Add1/1 -> Product3/1
  Gain2/1 -> Product1/1
  Tsc/1 -> Product2/2
  Q/1 -> Product5/2
  Gain1/1 -> Add2/1, Add1/1

== system Simulation/Motor Control and Resistance Estimation/Proposed method/Detect rising edge ==
  In : Inport
  Compare To Constant : simulink/Logic and Bit Operations/Compare To Constant  relop=>=  const=1  OutDataTypeStr=boolean
  Compare To Constant1 : simulink/Logic and Bit Operations/Compare To Constant  relop=<  const=1  OutDataTypeStr=boolean
  Logical Operator : Logic  AllPortsSameDT=off  OutDataTypeStr=boolean
  delay : UnitDelay  SampleTime=-1
  Out : Outport
  wires:
  delay/1 -> Compare To Constant1/1
  Logical Operator/1 -> Out/1
  In/1 -> Compare To Constant/1, delay/1
  Compare To Constant/1 -> Logical Operator/1
  Compare To Constant1/1 -> Logical Operator/2

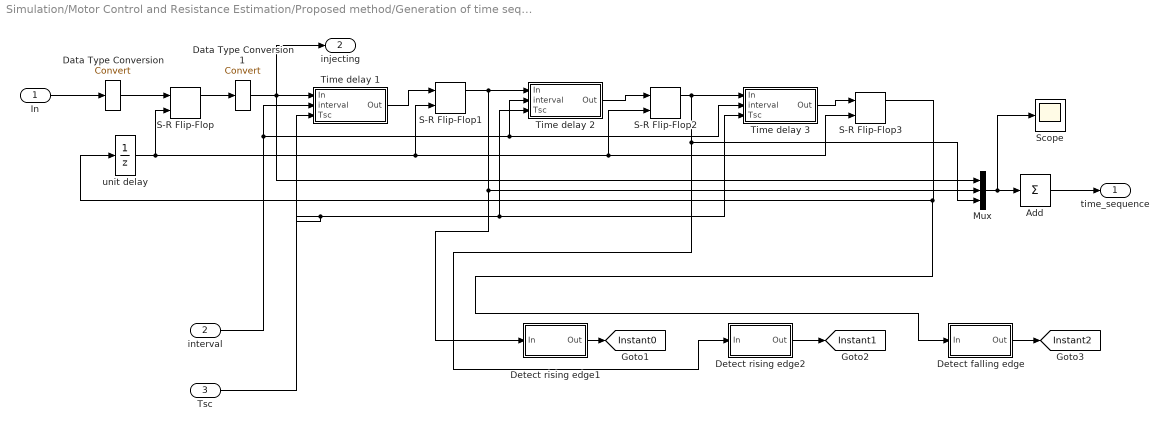
== system Simulation/Motor Control and Resistance Estimation/Proposed method/Generation of time sequence for injection ==
  In : Inport
  interval : Inport  Port=2
  Tsc : Inport  Port=3
  Add : Sum  Inputs=+
  Data Type Conversion : DataTypeConversion
  Data Type Conversion1 : DataTypeConversion
  Detect falling edge : Subsystem
  Detect rising edge1 : Subsystem
  Detect rising edge2 : Subsystem
  Mux : Mux  Inputs=3
  S-R Flip-Flop{,1..3} (4 alike) : simulink_extras/Flip Flops/S-R Flip-Flop  initial_condition=0
  Scope : Scope
  Time delay 1 : Subsystem
  Time delay 2 : Subsystem
  Time delay 3 : Subsystem
  unit delay : UnitDelay  SampleTime=-1
  time_sequence : Outport
  injecting : Outport  Port=2
  tag scope: Instant0=global, Instant1=global, Instant2=global
  wires:
  S-R Flip-Flop/1 -> Data Type Conversion1/1
  Data Type Conversion1/1 -> Mux/1, injecting/1, Time delay 1/1(In)
  S-R Flip-Flop1/1 -> Detect rising edge1/1(In), Mux/2, Time delay 2/1(In)
  Data Type Conversion/1 -> S-R Flip-Flop/1
  In/1 -> Data Type Conversion/1
  Time delay 1/1(Out) -> S-R Flip-Flop1/1
  S-R Flip-Flop3/1 -> Detect falling edge/1(In), unit delay/1
  Time delay 2/1(Out) -> S-R Flip-Flop2/1
  unit delay/1 -> S-R Flip-Flop3/2, S-R Flip-Flop2/2, S-R Flip-Flop1/2, S-R Flip-Flop/2
  S-R Flip-Flop2/1 -> Detect rising edge2/1(In), Mux/3, Time delay 3/1(In)
  Time delay 3/1(Out) -> S-R Flip-Flop3/1
  Mux/1 -> Scope/1, Add/1
  Add/1 -> time_sequence/1
  Detect rising edge1/1(Out) -> [Instant0]
  Detect rising edge2/1(Out) -> [Instant1]
  Detect falling edge/1(Out) -> [Instant2]
  interval/1 -> Time delay 3/2(interval), Time delay 2/2(interval), Time delay 1/2(interval)
  Tsc/1 -> Time delay 3/3(Tsc), Time delay 2/3(Tsc), Time delay 1/3(Tsc)

== system Simulation/Motor Control and Resistance Estimation/Proposed method/R estimation ==
  Vpk : Inport
  ws : Inport  Port=2
  NF_Q : Inport  Port=3
  LPF_BW : Inport  Port=4
  Tsc : Inport  Port=5
  Idc : Inport  Port=6
  Healthy/OPF : Inport  Port=7
  Equations (10) & (11) : Subsystem
  Low-pass filter : Subsystem
  Notch filter : Subsystem
  Subsystem : Subsystem
  "R " : Outport
  tag scope: filtered_vpk=global
  wires:
  LPF_BW/1 -> Low-pass filter/2(BW)  "Bandwidth of low-pass filter (rad/s)"
  Tsc/1 -> Notch filter/3(Tsc)  "Control sampling period"
  Low-pass filter/1(Out) -> Notch filter/1(In)
  NF_Q/1 -> Notch filter/4(Q)  "Quality factor of notch filter"
  ws/1 -> Notch filter/2(ws)  "Stator fundamental frequency (rad/s)"
  Vpk/1 -> Low-pass filter/1(Vpk)  "Pole voltages (V)"
  Notch filter/1(Out) -> Subsystem/1(In), Equations (10) & (11)/1(V)  "Filtered pole voltages (V)"
  Idc/1 -> Equations (10) & (11)/3(Idc)  "dc current magnitude (A)"
  Equations (10) & (11)/1(R) -> "R "/1
  Healthy/OPF/1 -> Subsystem/2(Healthy_OPF), Equations (10) & (11)/2(Healthy/OPF)
  Subsystem/1(Out) -> [filtered_vpk]

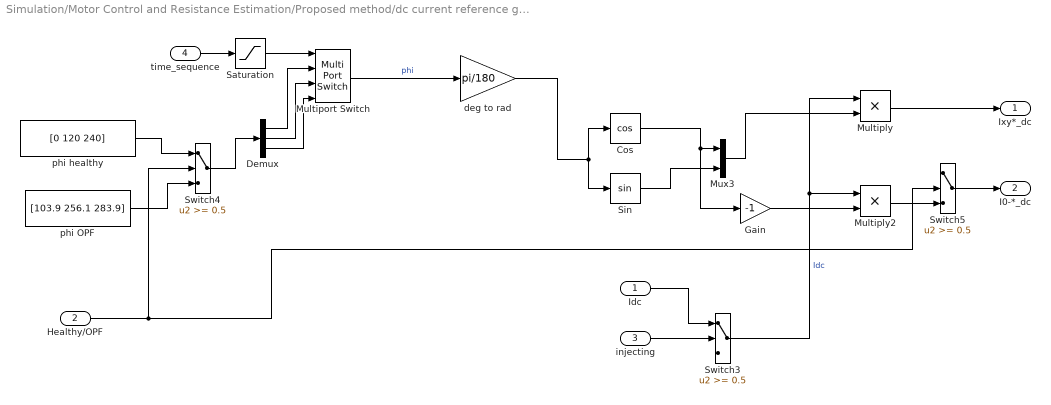
== system Simulation/Motor Control and Resistance Estimation/Proposed method/dc current reference generation ==
  Idc : Inport
  Healthy/OPF : Inport  Port=2
  injecting : Inport  Port=3
  time_sequence : Inport  Port=4
  Cos : Trigonometry  Operator=cos
  Demux : Demux  Outputs=3
  Gain : Gain  Gain=-1
  Multiply : Product
  Multiply2 : Product
  Multiport Switch : MultiPortSwitch
  Mux3 : Mux  Inputs=2
  Saturation : Saturate  UpperLimit=3  LowerLimit=1
  Sin : Trigonometry
  Switch3 : Switch  Threshold=0.5  SaturateOnIntegerOverflow=on
  Switch4 : Switch  Threshold=0.5  SaturateOnIntegerOverflow=on
  Switch5 : Switch  Threshold=0.5  SaturateOnIntegerOverflow=on
  deg to rad : Gain  Gain=pi/180
  phi OPF : Constant  Value=[103.9 256.1 283.9]
  phi healthy : Constant  Value=[0 120 240]
  Ixy*_dc : Outport
  I0-*_dc : Outport  Port=2
  wires:
  injecting/1 -> Switch3/2
  Sin/1 -> Mux3/2
  Cos/1 -> Gain/1, Mux3/1
  Mux3/1 -> Multiply/2
  Gain/1 -> Multiply2/2
  Multiply/1 -> Ixy*_dc/1
  Switch5/1 -> I0-*_dc/1
  Multiport Switch/1 -> deg to rad/1  "phi"
  Switch3/1 -> Multiply/1, Multiply2/1  "Idc"
  deg to rad/1 -> Cos/1, Sin/1
  Idc/1 -> Switch3/1
  phi healthy/1 -> Switch4/1
  Demux/1 -> Multiport Switch/2
  Demux/3 -> Multiport Switch/4
  Demux/2 -> Multiport Switch/3
  Switch4/1 -> Demux/1
  phi OPF/1 -> Switch4/3
  Healthy/OPF/1 -> Switch4/2, Switch5/2
  Multiply2/1 -> Switch5/3
  Saturation/1 -> Multiport Switch/1
  time_sequence/1 -> Saturation/1

== system Simulation/Motor Control and Resistance Estimation/Resonant controller 0-/Adaptive Impulse invariant ==
  in : Inport
  Wo : Inport  Port=2
  Divide : Product  Inputs=**
  Divide1 : Product  Inputs=**
  Gain : Gain  Gain=Tsc
  Gain1 : Gain  Gain=Tsc
  Gain3 : Gain  Gain=2
  Sum2 : Sum  Inputs=|+-|+-
  Trigonometric Function : Trigonometry  Operator=cos
  Unit Delay : UnitDelay  SampleTime=-1  HasFrameUpgradeWarning=on
  Unit Delay1 : UnitDelay  SampleTime=-1  HasFrameUpgradeWarning=on
  Unit Delay3 : UnitDelay  SampleTime=-1  HasFrameUpgradeWarning=on
  out : Outport
  wires:
  Unit Delay3/1 -> Sum2/4
  Wo/1 -> Gain1/1
  in/1 -> Gain/1
  Sum2/1 -> Unit Delay1/1, out/1
  Trigonometric Function/1 -> Divide1/2, Divide/2
  Divide/1 -> Unit Delay/1
  Unit Delay1/1 -> Unit Delay3/1, Divide1/1
  Divide1/1 -> Gain3/1
  Gain3/1 -> Sum2/3
  Gain/1 -> Sum2/1, Divide/1
  Gain1/1 -> Trigonometric Function/1
  Unit Delay/1 -> Sum2/2

== system Simulation/Motor Control and Resistance Estimation/Resonant controller ab/Adaptive Impulse invariant ==
  in : Inport
  Wo : Inport  Port=2
  Divide : Product  Inputs=**
  Divide1 : Product  Inputs=**
  Gain : Gain  Gain=Tsc
  Gain1 : Gain  Gain=Tsc
  Gain3 : Gain  Gain=2
  Sum2 : Sum  Inputs=|+-|+-
  Trigonometric Function : Trigonometry  Operator=cos
  Unit Delay : UnitDelay  SampleTime=-1  HasFrameUpgradeWarning=on
  Unit Delay1 : UnitDelay  SampleTime=-1  HasFrameUpgradeWarning=on
  Unit Delay3 : UnitDelay  SampleTime=-1  HasFrameUpgradeWarning=on
  out : Outport
  wires:
  Unit Delay3/1 -> Sum2/4
  Wo/1 -> Gain1/1
  in/1 -> Gain/1
  Sum2/1 -> Unit Delay1/1, out/1
  Trigonometric Function/1 -> Divide1/2, Divide/2
  Divide/1 -> Unit Delay/1
  Unit Delay1/1 -> Unit Delay3/1, Divide1/1
  Divide1/1 -> Gain3/1
  Gain3/1 -> Sum2/3
  Gain/1 -> Sum2/1, Divide/1
  Gain1/1 -> Trigonometric Function/1
  Unit Delay/1 -> Sum2/2

== system Simulation/Motor Control and Resistance Estimation/Resonant controller xy/Adaptive Impulse invariant ==
  in : Inport
  Wo : Inport  Port=2
  Divide : Product  Inputs=**
  Divide1 : Product  Inputs=**
  Gain : Gain  Gain=Tsc
  Gain1 : Gain  Gain=Tsc
  Gain3 : Gain  Gain=2
  Sum2 : Sum  Inputs=|+-|+-
  Trigonometric Function : Trigonometry  Operator=cos
  Unit Delay : UnitDelay  SampleTime=-1  HasFrameUpgradeWarning=on
  Unit Delay1 : UnitDelay  SampleTime=-1  HasFrameUpgradeWarning=on
  Unit Delay3 : UnitDelay  SampleTime=-1  HasFrameUpgradeWarning=on
  out : Outport
  wires:
  Unit Delay/1 -> Sum2/2
  Gain1/1 -> Trigonometric Function/1
  Gain/1 -> Divide/1, Sum2/1
  Gain3/1 -> Sum2/3
  Divide1/1 -> Gain3/1
  Unit Delay1/1 -> Divide1/1, Unit Delay3/1
  Divide/1 -> Unit Delay/1
  Trigonometric Function/1 -> Divide/2, Divide1/2
  Sum2/1 -> out/1, Unit Delay1/1
  in/1 -> Gain/1
  Wo/1 -> Gain1/1
  Unit Delay3/1 -> Sum2/4

== system Simulation/Motor Control and Resistance Estimation/Speed control loop/Subsystem2 ==
  Id* : Inport
  Iq* : Inport  Port=2
  wr : Inport  Port=3
  Estimation of rotor-flux position and speed : Subsystem
  Inverse Park transformation : Subsystem
  Mux2 : Mux  Inputs=2
  Iab : Outport  VectorParamsAs1DForOutWhenUnconnected=off
  ws : Outport  Port=2  VectorParamsAs1DForOutWhenUnconnected=off
  wires:
  Estimation of rotor-flux position and speed/2("ws ") -> ws/1
  Inverse Park transformation/1("Ia*, Ib*") -> Iab/1
  Mux2/1 -> Inverse Park transformation/1("Id*, Iq*")
  Id*/1 -> Mux2/1, Estimation of rotor-flux position and speed/1(Id*)
  wr/1 -> Estimation of rotor-flux position and speed/3(speed)
  Iq*/1 -> Mux2/2, Estimation of rotor-flux position and speed/2(Iq*)
  Estimation of rotor-flux position and speed/1(theta_r) -> Inverse Park transformation/2("theta_r ")
